simulink model "Sim_exercise2"  (R2015b)
settings: Solver=VariableStepAuto  StartTime=0.0  StopTime=10.0  RelTol=1e-3
undefined symbols (not defined in the file): A, A1, B, B1, C, C1, D, D1, dm, Jeq, Kemf, Km, n, R
settings Model: Creator=sofianh  LastModifiedBy=sofianh

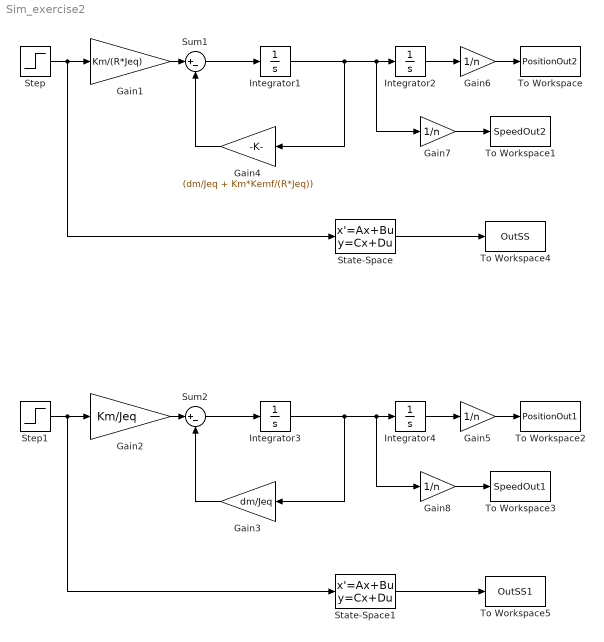
== system Sim_exercise2 ==
  Gain1 : Gain  Gain=Km/(R*Jeq)
  Gain2 : Gain  Gain=Km/Jeq
  Gain3 : Gain  Gain=dm/Jeq
  Gain4 : Gain  Gain=(dm/Jeq + Km*Kemf/(R*Jeq))
  Gain{5..8} (4 alike) : Gain  Gain=1/n
  Integrator{1..4} (4 alike) : Integrator
  State-Space : StateSpace  A=A  B=B  C=C  D=D  X0=0  ContinuousStateAttributes='Position'
  State-Space1 : StateSpace  A=A1  B=B1  C=C1  D=D1  X0=0  ContinuousStateAttributes='Position'
  Step : Step  Time=0  SampleTime=0
  Step1 : Step  Time=0  SampleTime=0
  Sum1 : Sum  Inputs=|+-
  Sum2 : Sum  Inputs=|+-
  To Workspace : ToWorkspace  VariableName=PositionOut2  SaveFormat=Structure With Time  SampleTime=-1
  To Workspace1 : ToWorkspace  VariableName=SpeedOut2  SaveFormat=Structure With Time  SampleTime=-1
  To Workspace2 : ToWorkspace  VariableName=PositionOut1  SaveFormat=Structure With Time  SampleTime=-1
  To Workspace3 : ToWorkspace  VariableName=SpeedOut1  SaveFormat=Structure With Time  SampleTime=-1
  To Workspace4 : ToWorkspace  VariableName=OutSS  SaveFormat=Structure With Time  SampleTime=-1
  To Workspace5 : ToWorkspace  VariableName=OutSS1  SaveFormat=Structure With Time  SampleTime=-1
  wires:
  State-Space/1 -> To Workspace4/1
  Step/1 -> Gain1/1, State-Space/1
  Sum1/1 -> Integrator1/1
  Integrator1/1 -> Gain4/1, Gain7/1, Integrator2/1
  Gain4/1 -> Sum1/2
  Integrator2/1 -> Gain6/1
  Gain6/1 -> To Workspace/1
  Gain7/1 -> To Workspace1/1
  Gain1/1 -> Sum1/1
  State-Space1/1 -> To Workspace5/1
  Step1/1 -> Gain2/1, State-Space1/1
  Sum2/1 -> Integrator3/1
  Integrator3/1 -> Gain3/1, Gain8/1, Integrator4/1
  Gain3/1 -> Sum2/2
  Integrator4/1 -> Gain5/1
  Gain5/1 -> To Workspace2/1
  Gain8/1 -> To Workspace3/1
  Gain2/1 -> Sum2/1
